simulink model "mpc_model_alignment"  (R2019a)
settings: Solver=FixedStepAuto  StartTime=0.0  StopTime=Tfinal  RelTol=1e-3
values from neighbouring files (symbols this model uses):
  A = [-0.0285 -0.0014; -0.0371 -0.1476]    [model.m]
  AlignmentPeriod = 0.5    [mpc_model_parameters.m]
  DCLINK_Cap = 1000e-12    (= 1e-09)    [mpc_model_parameters.m]    (also in mpc_model_parameters_dual_module.m = 0.001)
  FaultTime = 50    [mpc_model_parameters.m]
  FluxPM = MeanInducedVoltagePeak/(2*pi*100)    [mpc_model_parameters.m]    (also in mpc_model_parameters_dual_module.m)
  Fsw_Alignment = 10000    [mpc_model_parameters.m]
  Inertia = 1e-2    (= 0.01)    [mpc_model_parameters.m]    (also in mpc_model_parameters_dual_module.m)
  Ls = 3.5e-3    (= 0.0035)    [MPC_id_iq.m]    (also in mpc_model_parameters.m = 0.00351; mpc_model_parameters_dual_module.m = 0.00343)
  PolePairs = 10    [mpc_model_parameters.m]    (also in mpc_model_parameters_dual_module.m)
  Rin = 1e-3    (= 0.001)    [mpc_model_parameters.m]    (also in mpc_model_parameters_dual_module.m)
  Rs = 0.531    [Loss_Distribution.m]    (also in MPC_id_iq.m; mpc_model_parameters.m = 0.321; mpc_model_parameters_dual_module.m = 0.539)
  Sampling_time = 1e-6    (= 1e-06)    [mpc_model_parameters.m]    (also in mpc_model_parameters_dual_module.m)
  SpeedRef1 = 0    [mpc_model_parameters.m]    (also in mpc_model_parameters_dual_module.m = 35)
  SpeedRef2 = 50    [mpc_model_parameters.m]    (also in mpc_model_parameters_dual_module.m = 35)
  SpeedRefUpdateTime = 0.5    [mpc_model_parameters.m]    (also in mpc_model_parameters_dual_module.m = 1.75)
  Tload1 = 0    [mpc_model_parameters.m]    (also in mpc_model_parameters_dual_module.m = 30)
  Tload2 = 20    [mpc_model_parameters.m]    (also in mpc_model_parameters_dual_module.m = 63.6619772368)
  TloadUpdateTime = 0.6    [mpc_model_parameters.m]    (also in mpc_model_parameters_dual_module.m = 0.5)
  Vdc = 30    [mpc_model_parameters.m]    (also in mpc_model_parameters_dual_module.m = 40)
  Vin = Vdc + Rin*(Pout/Vdc)    (= 30.0666666667)    [mpc_model_parameters.m]    (also in mpc_model_parameters_dual_module.m = 40.05)
  ViscousFriction = 1e-3    (= 0.001)    [mpc_model_parameters.m]    (also in mpc_model_parameters_dual_module.m)
  whitenoisegain = 0    [mpc_model_parameters.m]
undefined symbols (not defined in the file or in its folder): DiscIntNeverNeededParam
libraries: powerlib x16, dspswit3 x7, simulink x4, powerlib_meascontrol x3, dspstat3 x3, dspsigops x1
settings Model: Creator=hakan  LastModifiedBy=hakan
settings SolverCC: ZeroCrossAlgorithm=Adaptive
settings DebuggingCC: IgnoredZcDiagnostic=none

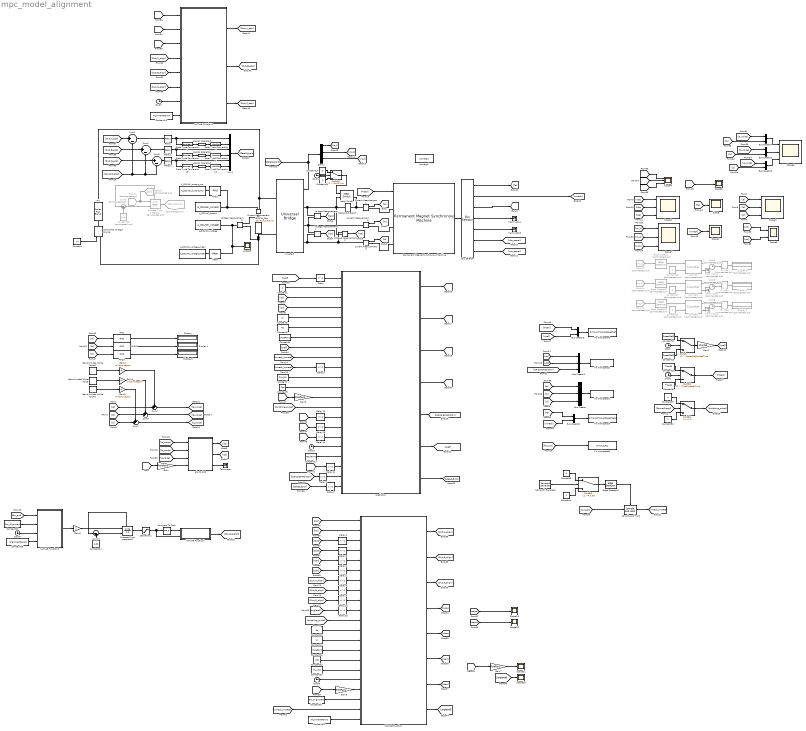
== system mpc_model_alignment ==
  A_DCLINK_current : ToWorkspace  VariableName=A_DCLINK_current  SaveFormat=Structure With Time  SampleTime=-1
  A_DCLINK_current_rms : ToWorkspace  VariableName=A_DCLINK_current_rms  SaveFormat=Structure With Time  SampleTime=-1
  A_DCLINK_voltage : ToWorkspace  VariableName=A_DCLINK_voltage  SaveFormat=Structure With Time  SampleTime=-1
  A_DCLINK_voltage_mean : ToWorkspace  VariableName=A_DCLINK_voltage_mean  SaveFormat=Structure With Time  SampleTime=-1
  Band-Limited White Noise : simulink/Sources/Band-Limited White Noise  Cov=[0.00000002]  Ts=Sampling_time  seed=[23344]  VectorParams1D=off
  Band-Limited White Noise1 : simulink/Sources/Band-Limited White Noise  Cov=[0.00000002]  Ts=Sampling_time  seed=[23343]  VectorParams1D=off
  Band-Limited White Noise2 : simulink/Sources/Band-Limited White Noise  Cov=[0.00000002]  Ts=Sampling_time  seed=[23341]  VectorParams1D=off
  Bus Creator : BusCreator  Inputs=3
  Bus Creator1 : BusCreator  Inputs=3
  Bus Creator{2..6} (5 alike) : BusCreator  Inputs=2
  Bus Selector : BusSelector  OutputSignals=Electromagnetic torque Te (N*m),Rotor speed wm (rad/s),Rotor angle thetam (rad),Stator current is_q (A),Stator current is_d (A),Stator voltage Vs_q (V),Stator voltage Vs_d (V)
  Clock{,1..3,7..9} (7 alike) : Clock
  Clock4 : Clock  Commented=on
  Clock5 : Clock  Commented=on
  Clock6 : Clock  Commented=on
  Compare To Zero : simulink/Logic and Bit Operations/Compare To Zero  relop===  OutDataTypeStr=boolean
  Constant : Constant  Value=Vin
  Constant{1,3,15,29} (4 alike) : Constant  Value=0
  Constant10 : Constant  Value=SpeedRef1
  Constant11 : Constant  Value=SpeedRef2
  Constant12 : Constant  Value=Tload2
  Constant13 : Constant  Value=AlignmentPeriod
  Constant14 : Constant  Value=Ls
  Constant16 : Constant
  Constant17 : Constant  Value=FaultTime
  Constant18 : Constant  Commented=on  Value=0
  Constant19 : Constant  Commented=on  Value=0
  Constant2 : Constant  Value=Ls
  Constant20 : Constant  Commented=on  Value=0
  Constant21 : Constant  Value=Rs
  Constant22 : Constant  Value=PolePairs
  Constant23 : Constant  Value=Vdc
  Constant24 : Constant  Value=1.02
  Constant25 : Constant  Value=AlignmentPeriod
  Constant26 : Constant  Commented=on  Value=1.04
  Constant27 : Constant  Value=Fsw_Alignment
  Constant28 : Constant  Value=AlignmentPeriod
  Constant30 : Constant
  Constant31 : Constant  Value=Fsw_Alignment
  Constant32 : Constant  Value=FluxPM
  Constant4 : Constant
  Constant5 : Constant  Value=Rs
  Constant6 : Constant  Value=PolePairs
  Constant7 : Constant  Value=FluxPM
  Constant8 : Constant  Value=Tload1
  Constant9 : Constant  Value=Vdc
  Controlled Voltage Source : powerlib/Electrical Sources/Controlled Voltage Source  Initialize=on  Source_Type=DC  Amplitude=Vin  Phase=0  Frequency=0  Measurements=None
      settings: SourceProductName=Simscape Electrical
  Counter : dspswit3/Counter  Commented=on  Direction=Up  CountEvent=Rising edge  CounterSize=User defined  MaxCount=9999999999999999999  InitialCount=0  Output=Count and Hit  HitValue=32  ResetInput=on  SamplesPerFrame=1  Ts=1  CntDtype=double  HitDtype=Logical
  Counter1 : dspswit3/Counter  Commented=on  Direction=Up  CountEvent=Rising edge  CounterSize=User defined  MaxCount=9999999999999999999  InitialCount=0  Output=Count and Hit  HitValue=32  ResetInput=on  SamplesPerFrame=1  Ts=1  CntDtype=double  HitDtype=Logical
  Counter2 : dspswit3/Counter  Commented=on  Direction=Up  CountEvent=Rising edge  CounterSize=User defined  MaxCount=9999999999999999999  InitialCount=0  Output=Count and Hit  HitValue=32  ResetInput=on  SamplesPerFrame=1  Ts=1  CntDtype=double  HitDtype=Logical
  Current Measurement{,1..3} (4 alike) : powerlib/Measurements/Current Measurement  PhasorSimulation=off  OutputType=Complex  PSBequivalent=0
      settings: SourceProductName=Simscape Electrical
  DCLINK_Cap : powerlib/Elements/Series RLC Branch  LConnTagsString=__new0  RConnTagsString=__new0  BranchType=C  Resistance=1  Inductance=1e-3  SetiL0=off  InitialCurrent=0  Capacitance=DCLINK_Cap  Setx0=on  InitialVoltage=Vin  Measurements=None
      settings: SourceProductName=Simscape Electrical
  Data Type Conversion10 : DataTypeConversion  OutDataTypeStr=boolean
  Data Type Conversion11 : DataTypeConversion  OutDataTypeStr=double
  Data Type Conversion6 : DataTypeConversion  OutDataTypeStr=boolean
  Data Type Conversion7 : DataTypeConversion  OutDataTypeStr=double
  Data Type Conversion8 : DataTypeConversion  OutDataTypeStr=boolean
  Data Type Conversion9 : DataTypeConversion  OutDataTypeStr=double
  Delay{,1..15} (16 alike) : Delay  DelayLength=1
  Demux : Demux  Outputs=6
  Discrete-Time Integrator : DiscreteIntegrator  Commented=on  ExternalReset=falling  SampleTime=-1  ShowStatePort=on  ICPrevOutput=DiscIntNeverNeededParam  ICPrevScaledInput=DiscIntNeverNeededParam
  Discrete-Time Integrator2 : DiscreteIntegrator  ExternalReset=falling  SampleTime=Sampling_time  UpperSaturationLimit=1  LowerSaturationLimit=0  ShowStatePort=on  ICPrevOutput=DiscIntNeverNeededParam  ICPrevScaledInput=DiscIntNeverNeededParam
  Display : Display
  Display1 : Display  Commented=on
  Display2 : Display  Commented=on
  Display3 : Display  Commented=on
  Display4 : Display
  Display5 : Display
  Divide : Product  Commented=on  Inputs=*/
  Divide1 : Product  Commented=on  Inputs=*/
  Divide2 : Product  Commented=on  Inputs=*/
  Edge Detector : dspswit3/Edge Detector  Commented=on  InputProcessing=Columns as channels (frame based)
      settings: SourceProductName=DSP System Toolbox  SourceProductBaseCode=DS
  Edge Detector1 : dspswit3/Edge Detector  Commented=on  InputProcessing=Columns as channels (frame based)
      settings: SourceProductName=DSP System Toolbox  SourceProductBaseCode=DS
  Edge Detector2 : dspswit3/Edge Detector  Commented=on  InputProcessing=Columns as channels (frame based)
      settings: SourceProductName=DSP System Toolbox  SourceProductBaseCode=DS
  Edge Detector3 : dspswit3/Edge Detector  InputProcessing=Columns as channels (frame based)
      settings: SourceProductName=DSP System Toolbox  SourceProductBaseCode=DS
  From40 : From  Commented=on  GotoTag=va_1
  From41 : From  Commented=on  GotoTag=vb_1
  From42 : From  Commented=on  GotoTag=vc_1
  From72 : From  Commented=on  GotoTag=fsw_out
  Gain{,3,6..7} (4 alike) : Gain  Gain=PolePairs
  Gain1 : Gain  Gain=2*pi/60
  Gain2 : Gain  Gain=whitenoisegain
  Gain4 : Gain  Gain=whitenoisegain
  Gain5 : Gain  Gain=whitenoisegain
  Gain8 : Gain  Gain=2
  Goto29 : Goto  Commented=on  GotoTag=fsw
  Goto9 : Goto  Commented=on  GotoTag=CarrierSignal
  Ideal Switch : powerlib/Power Electronics/Ideal Switch  Ron=0.001  Lon=0  IC=0  Rs=1e5  Cs=inf  Measurements=on
      settings: SourceProductName=Simscape Electrical
  Inverter1 : powerlib/Power Electronics/Universal Bridge  Arms=3  SnubberResistance=1e5  SnubberCapacitance=inf  Device=IGBT / Diodes  Ron=0.65e-3  Lon=0  ForwardVoltages="[  0  0  ]"  ForwardVoltage=0  GTOparameters=[ 10e-6 , 20e-6 ]  IGBTparameters=[ 1e-6 , 2e-6 ]  Measurements=All voltages and currents  Measurements_2=None  converterType=Rectifier
      settings: SourceProductName=Simscape Electrical
  Logical Operator3 : Logic  Operator=NOT  AllPortsSameDT=off  OutDataTypeStr=boolean
  Logical Operator4 : Logic  Operator=NOT  AllPortsSameDT=off  OutDataTypeStr=boolean
  Logical Operator5 : Logic  Operator=NOT  AllPortsSameDT=off  OutDataTypeStr=boolean
  MATLAB Function : MATLAB Function  TreatAsAtomicUnit=on
  MATLAB Function1 : MATLAB Function  TreatAsAtomicUnit=on
  MATLAB Function2 : MATLAB Function  TreatAsAtomicUnit=on
  MATLAB Function3 : MATLAB Function  TreatAsAtomicUnit=on
  Mean : powerlib_meascontrol/Measurements/Mean  Freq=THD_mean_frequency  Vinit=0  Ts=0
      settings: SourceProductName=Simscape Electrical
  Mux4 : Mux  Inputs=6
  Permanent Magnet Synchronous Machine : powerlib/Machines/Permanent Magnet Synchronous Machine  NbPhases=3  FluxDistribution=Sinusoidal  RotorType=Round  MechanicalLoad=Torque Tm  PresetModel=No  ShowDetailedParameters=on  MeasurementBus=off  Resistance=Rs  Inductance=8.5e-3  dqInductances=[3.1e-3,3.6e-3]  La=Ls  MachineConstant=Voltage Constant (V_peak L-L / krpm)  Flux=0.18074  VoltageCst=VoltageConstant  TorqueCst=2.7111  Flat=120  Mechanical=[Inertia ViscousFriction PolePairs 0]  PolePairs=4  InitialConditions=[0*100*2*pi/60,0, 0,0]  InitialConditions5ph=[0 0 0 0 0 0]  TsPowergui=0  TsBlock=-1  RefAngle=90 degrees behind phase A axis (modified Park)
  RMS : dspstat3/RMS  run=off  directionMode=Each column  dimension=1  InputProcessing=Columns as channels (frame based)  reset_popup=None
  RMS1 : powerlib_meascontrol/Measurements/RMS  TrueRMS=on  Freq=Load_Nominal_Freq  RMSInit=10  Ts=0
      settings: SourceProductName=Simscape Electrical
  RMS2 : dspstat3/RMS  run=off  directionMode=Each column  dimension=1  InputProcessing=Columns as channels (frame based)  reset_popup=None
  RMS3 : dspstat3/RMS  run=off  directionMode=Each column  dimension=1  InputProcessing=Columns as channels (frame based)  reset_popup=None
  Relay : Relay
  Relay1 : Relay
  Relay2 : Relay
  Rin : powerlib/Elements/Series RLC Branch  LConnTagsString=__new0  RConnTagsString=__new0  BranchType=R  Resistance=Rin  Inductance=1e-3  SetiL0=off  InitialCurrent=0  Capacitance=1000e-6  Setx0=off  InitialVoltage=0  Measurements=None
      settings: SourceProductName=Simscape Electrical
  Sample and Hold : dspsigops/Sample and Hold  trig=Rising edge  initCond=0  latchinput=off
  Saturation1 : Saturate  UpperLimit=1  LowerLimit=0
  Sawtooth Generator : powerlib_meascontrol/Pulse & Signal Generators/Sawtooth Generator  Freq=100  Phase=180  Ts=0
      settings: SourceProductName=Simscape Electrical
  Scope{,1,5,9..13} (8 alike) : Scope
  Scope{2..4,6..7} (5 alike) : Scope  NumInputPorts=3
  Scope8 : Scope  NumInputPorts=2
  Series RLC Branch : powerlib/Elements/Series RLC Branch  LConnTagsString=__new0  RConnTagsString=__new0  BranchType=R  Resistance=5000  Inductance=1e-3  SetiL0=off  InitialCurrent=0  Capacitance=1e-6  Setx0=off  InitialVoltage=0  Measurements=None
      settings: SourceProductName=Simscape Electrical
  Sum1 : Sum  Inputs=|+-
  Sum10 : Sum  Inputs=|-+
  Sum2 : Sum  Inputs=|+-
  Sum3 : Sum  Commented=on  Inputs=|-+
  Sum4 : Sum  Inputs=++|
  Sum5 : Sum  Inputs=|+-
  Sum6 : Sum  Inputs=++|
  Sum7 : Sum  Inputs=++|
  Switch : Switch  Criteria=u2 > Threshold  Threshold=SpeedRefUpdateTime
  Switch1 : Switch  Criteria=u2 > Threshold  Threshold=TloadUpdateTime
  Switch2 : Switch  Threshold=0.99
  Switch3 : Switch  Criteria=u2 > Threshold  Threshold=FaultTime
  Switch4 : Switch  Criteria=u2 ~= 0
  Terminator : Terminator
  Terminator1 : Terminator  Commented=on
  Terminator2 : Terminator  Commented=on
  Terminator3 : Terminator  Commented=on
  Terminator4 : Terminator
  Terminator5 : Terminator
  To Workspace1 : ToWorkspace  VariableName=Simout_PhaseCurrents_abc  SaveFormat=Timeseries  SampleTime=-1
  To Workspace2 : ToWorkspace  VariableName=Simout_PhaseCurrents_dq  SaveFormat=Timeseries  SampleTime=-1
  To Workspace3 : ToWorkspace  VariableName=Simout_TorqueSpeedMeas  SaveFormat=Timeseries  SampleTime=-1
  To Workspace4 : ToWorkspace  VariableName=Simout_TorqueSpeedRef  SaveFormat=Timeseries  SampleTime=-1
  To Workspace5 : ToWorkspace  VariableName=Simout_Fsw  SaveFormat=Timeseries  SampleTime=-1
  Voltage Measurement{,1..3} (4 alike) : powerlib/Measurements/Voltage Measurement  PhasorSimulation=off  OutputType=Complex  PSBequivalent=0
      settings: SourceProductName=Simscape Electrical
  abc to dq0 : MATLAB Function  TreatAsAtomicUnit=on
  powergui : powerlib/powergui  Priority=1  SimulationMode=Discrete  SampleTime=Sampling_time  frequency=60  Iterations=50  frequencyindice=0  Pbase=100e6  ErrMax=1e-4  UnitsV=kV  UnitsW=MW  buscounter=0  FunctionMessages=off  echomessages=off  EnableUseOfTLC=off  CurrentSourceSwitches=off  DisableSnubberDevices=off  DisableRonSwitches=off  DisableVfSwitches=off  DisplayEquations=off  AutomaticDiscreteSolvers=off  SolverType=Tustin/Backward Euler (TBE)  Interpol=off  ExternalGateDelay=off  methode=off  Ts=100  x0status=blocks  SPID=on  SwTol=0  HookPort=off  NonlinearTolerance=0  nMaxIteration=15  ContinueOnMaxIteration=off  RestoreLinks=warning  ResistiveCurrentMeasurement=off  Frange=[0:2:500]  Ylog=off  Xlog=on  ShowGrid=off  save=off  variable=ZData  structure=0  ZoomFFT=off  StartTime=0.0  cycles=1  DisplayStyle=1  fundamental=60  FreqAxis=off  MaxFrequency=1000  frequencyindicesteady=1  RmsSteady=1  display=off
      settings: SourceProductName=Simscape Electrical
  prediction : MATLAB Function  TreatAsAtomicUnit=on
  wires:
  Voltage Measurement3/1 -> Scope9/1, Mean/1, A_DCLINK_voltage/1
  RMS1/1 -> A_DCLINK_current_rms/1
  Constant/1 -> Controlled Voltage Source/1
  Mean/1 -> A_DCLINK_voltage_mean/1
  Current Measurement/1 -> RMS1/1, A_DCLINK_current/1
  Permanent Magnet Synchronous Machine/1 -> Bus Selector/1
  Bus Selector/1 -> [Te]  "<Electromagnetic torque Te (N*m)>"
  Bus Selector/2 -> [wmech]  "<Rotor speed wm (rad/s)>"
  Current Measurement1/1 -> [Ia]
  Current Measurement2/1 -> [Ib]
  Current Measurement3/1 -> [Ic]
  Bus Selector/3 -> [thetam]  "<Rotor angle thetam (rad)>"
  Bus Selector/4 -> Terminator4/1  "<Stator current is_q (A)>"
  Bus Selector/5 -> Terminator5/1  "<Stator current is_d (A)>"
  [ids] -> prediction/3(IdMeasured)
  [iqs] -> prediction/4(IqMeasured)
  Constant2/1 -> prediction/5(Ls)
  Voltage Measurement/1 -> [Vab]
  Voltage Measurement1/1 -> [Vbc]
  Voltage Measurement2/1 -> [Vca]
  Bus Selector/6 -> [vsq_actual]  "<Stator voltage Vs_q (V)>"
  Bus Selector/7 -> [vsd_actual]  "<Stator voltage Vs_d (V)>"
  [Vca] -> Scope2/3
  [Vbc] -> Scope2/2
  [Vab] -> Scope2/1
  Constant5/1 -> prediction/6(Rs)
  Constant6/1 -> prediction/7(PolePairs)
  [wmech_lowrate] -> prediction/9(ShaftAngularSpeed)
  Constant7/1 -> prediction/11(FluxPM)
  Constant9/1 -> prediction/12(Vdc)
  Gain3/1 -> prediction/13(ElectricalAngle)
  [thetam] -> Gain3/1
  [Tload] -> Permanent Magnet Synchronous Machine/1
  [iqs] -> Bus Creator1/2  "iqs"
  [ids] -> Bus Creator1/1  "ids"
  Constant10/1 -> Switch/3
  Constant11/1 -> Switch/1
  Switch/1 -> Gain1/1
  Clock/1 -> Switch/2
  Clock1/1 -> Switch1/2
  Constant12/1 -> Switch1/1
  Constant8/1 -> Switch1/3
  Switch1/1 -> [Tload]
  Bus Creator/1 -> To Workspace1/1  "Iabc"
  Bus Creator1/1 -> To Workspace2/1  "Idq"
  Bus Creator2/1 -> To Workspace3/1
  Gain1/1 -> [wref]
  [Tload] -> Bus Creator3/1  "Tload"
  [wref] -> Bus Creator3/2  "wref"
  Bus Creator3/1 -> To Workspace4/1
  [switching_pulse] -> prediction/14(InterruptPulse)
  Clock2/1 -> Switch3/2
  Constant15/1 -> Switch3/1
  Constant16/1 -> Switch3/3
  Switch3/1 -> Ideal Switch/1
  Clock3/1 -> prediction/18(SimulationClock)
  Constant17/1 -> prediction/19(FaultOccuranceTime)
  [va_1] -> Scope7/1
  [vb_1] -> Scope7/2
  [vc_1] -> Scope7/3
  Edge Detector/1 -> Counter/1
  Constant18/1 -> Counter/2
  Counter/1 -> Divide/1
  Clock4/1 -> Divide/2
  Divide/1 -> Display2/1
  [Ib] -> Bus Creator/2  "Ib"
  [Ia] -> Bus Creator/1  "Ia"
  [Ic] -> Bus Creator/3  "Ic"
  [Ib] -> Scope3/2  "Ib"
  [Ic] -> Scope3/3  "Ic"
  [Ia] -> Scope3/1  "Ia"
  [iqs] -> Scope8/1  "iqs"
  [ids] -> Scope8/2  "ids"
  Counter/2 -> Terminator1/1
  From40/1 -> Edge Detector/1
  From41/1 -> Edge Detector1/1
  Counter1/2 -> Terminator2/1
  Divide1/1 -> Display1/1
  Clock5/1 -> Divide1/2
  Counter1/1 -> Divide1/1
  Constant19/1 -> Counter1/2
  Edge Detector1/1 -> Counter1/1
  Edge Detector2/1 -> Counter2/1
  Constant20/1 -> Counter2/2
  Counter2/1 -> Divide2/1
  Clock6/1 -> Divide2/2
  Divide2/1 -> Display3/1
  Counter2/2 -> Terminator3/1
  From42/1 -> Edge Detector2/1
  [Te] -> Bus Creator2/1  "Te"
  [wmech] -> Bus Creator2/2  "wmech"
  [Te] -> Scope/1
  [wmech] -> Scope1/1
  prediction/1(DutyA) -> [DutyA]
  prediction/3(DutyC) -> [DutyC]
  prediction/2(DutyB) -> [DutyB]
  [DutyB] -> Scope4/2
  [DutyA] -> Scope4/1
  [DutyC] -> Scope4/3
  Constant26/1 -> Sum3/2
  From72/1 -> Goto29/1, Discrete-Time Integrator/1
  Discrete-Time Integrator/State -> Sum3/1
  Sum3/1 -> Discrete-Time Integrator/2
  Switch4/1 -> [switching_pulse]
  Constant30/1 -> Switch4/3
  Constant29/1 -> Switch4/1
  [GateSignals] -> Inverter1/1, Demux/1
  Demux/1 -> [va_1]
  Demux/3 -> [vb_1]
  prediction/4(FswSelected) -> [fsw_out]
  Delay11/1 -> prediction/20(FswSelected_prev)
  [fsw_out] -> Delay11/1
  [DutyB] -> Delay13/1
  [DutyA] -> Delay12/1
  [DutyC] -> Delay14/1
  Delay13/1 -> prediction/16(DutyB_prev)
  Delay12/1 -> prediction/15(DutyA_prev)
  Delay14/1 -> prediction/17(DutyC_prev)
  Discrete-Time Integrator/1 -> Goto9/1
  [CarrierSignal] -> Switch4/2
  Demux/5 -> [vc_1]
  [IqRipplePrediction] -> Delay1/1
  Delay1/1 -> prediction/21(IqRipplePrediction_prev)
  [CarrierSignal] -> Sum1/2, Sum2/2, Sum5/2
  Logical Operator4/1 -> Data Type Conversion9/1
  [DutyA_app] -> Sum1/1
  Data Type Conversion8/1 -> Logical Operator4/1
  Data Type Conversion10/1 -> Logical Operator5/1
  Relay1/1 -> Data Type Conversion8/1, Mux4/3
  Relay2/1 -> Data Type Conversion10/1, Mux4/5
  Data Type Conversion6/1 -> Logical Operator3/1
  Sum1/1 -> Relay/1
  Data Type Conversion11/1 -> Mux4/6
  [DutyC_app] -> Sum5/1
  Relay/1 -> Mux4/1, Data Type Conversion6/1
  Data Type Conversion9/1 -> Mux4/4
  Sum5/1 -> Relay2/1
  Logical Operator3/1 -> Data Type Conversion7/1
  Logical Operator5/1 -> Data Type Conversion11/1
  Sum2/1 -> Relay1/1
  Mux4/1 -> [GateSignals]
  [DutyB_app] -> Sum2/1
  Data Type Conversion7/1 -> Mux4/2
  [fsw_out] -> Scope5/1
  Discrete-Time Integrator2/State -> Sum10/1
  Gain8/1 -> Discrete-Time Integrator2/1
  Sum10/1 -> Discrete-Time Integrator2/2
  Saturation1/1 -> MATLAB Function1/2(inputwave), Compare To Zero/1
  Constant24/1 -> Sum10/2
  Discrete-Time Integrator2/1 -> Saturation1/1
  Compare To Zero/1 -> MATLAB Function1/1(pulse)
  MATLAB Function1/1(outputwave) -> [CarrierSignal]
  [fsw_out] -> To Workspace5/1
  [IqRipplePrediction] -> Bus Creator1/3  "iqripple"
  Constant1/1 -> prediction/2(idref)
  prediction/5(IqRipplePrediction) -> [IqRipplePrediction]
  Switch2/1 -> Edge Detector3/1
  Edge Detector3/1 -> Sample and Hold/Trigger
  Constant4/1 -> Switch2/3
  Sawtooth Generator/1 -> Switch2/2
  Constant3/1 -> Switch2/1
  [wmech] -> Sample and Hold/1
  Sample and Hold/1 -> [wmech_lowrate]
  [Ia] -> RMS/1
  [Ib] -> RMS2/1
  [Ic] -> RMS3/1
  RMS/1 -> Display/1
  RMS2/1 -> Display4/1
  RMS3/1 -> Display5/1
  abc to dq0/2(iqs) -> [iqs]
  Gain/1 -> abc to dq0/4(ref_frame_position)
  abc to dq0/1(ids) -> [ids]
  abc to dq0/3(i0) -> Terminator/1
  [thetam] -> Gain/1
  Sum4/1 -> [Ia_noise]
  [Ia] -> Sum4/2
  Sum6/1 -> [Ib_noise]
  [Ib] -> Sum6/2
  Sum7/1 -> [Ic_noise]
  [Ic] -> Sum7/2
  Band-Limited White Noise1/1 -> Gain5/1
  Band-Limited White Noise/1 -> Gain4/1
  Band-Limited White Noise2/1 -> Gain2/1
  Gain2/1 -> Sum4/1
  Gain4/1 -> Sum6/1
  Gain5/1 -> Sum7/1
  [Ia_noise] -> abc to dq0/1(ias)
  [Ib_noise] -> abc to dq0/2(ibs)
  [Ic_noise] -> abc to dq0/3(ics)
  [Ia_noise] -> Bus Creator4/1  "Ia_noise"
  [Ia] -> Bus Creator4/2  "Ia"
  [Ib] -> Bus Creator5/2  "Ib"
  [Ib_noise] -> Bus Creator5/1  "Ib_noise"
  [Ic_noise] -> Bus Creator6/1  "Ic_noise"
  [Ic] -> Bus Creator6/2  "Ic"
  Bus Creator5/1 -> Scope6/2
  Bus Creator4/1 -> Scope6/1
  Bus Creator6/1 -> Scope6/3
  prediction/6(iqref) -> [iqref]
  Delay/1 -> prediction/1(iqref_prev)
  [iqref] -> Delay/1
  [wref] -> prediction/8(wref)
  [wmech_lowrate] -> Delay3/1
  prediction/7(Speed_Error) -> [Speed_Error]
  Delay2/1 -> prediction/22(Speed_Error_prev)
  [Speed_Error] -> Delay2/1
  Delay3/1 -> prediction/10(ShaftAngularSpeed_prev)
  MATLAB Function/4(iqapp) -> [iqapp]
  MATLAB Function/5(idapp) -> [idapp]
  MATLAB Function/6(iqerr) -> [iqerr]
  MATLAB Function/7(iderr) -> [iderr]
  [iqapp] -> Delay4/1
  [idapp] -> Delay5/1
  [iqerr] -> Delay6/1
  [iderr] -> Delay7/1
  MATLAB Function/1(DutyA_align) -> [DutyA_align]
  MATLAB Function/2(DutyB_align) -> [DutyB_align]
  MATLAB Function/3(DutyC_align) -> [DutyC_align]
  [DutyA_align] -> Delay8/1
  [DutyB_align] -> Delay9/1
  [DutyC_align] -> Delay10/1
  [switching_pulse] -> MATLAB Function/11(InterruptPulse)
  [iqs] -> MATLAB Function/1(iqmeas)
  [ids] -> MATLAB Function/2(idmeas)
  [DutyA_align] -> MATLAB Function2/4(DutyA_align)
  [DutyC] -> MATLAB Function2/3(DutyC)
  [DutyB] -> MATLAB Function2/2(DutyB)
  [DutyA] -> MATLAB Function2/1(DutyA)
  [DutyB_align] -> MATLAB Function2/5(DutyB_align)
  [DutyC_align] -> MATLAB Function2/6(DutyC_align)
  Clock7/1 -> MATLAB Function2/7(clock)
  Constant13/1 -> MATLAB Function2/8(AlignmentPeriod)
  MATLAB Function2/1(DutyA_app) -> [DutyA_app]
  MATLAB Function2/3(DutyC_app) -> [DutyC_app]
  MATLAB Function2/2(DutyB_app) -> [DutyB_app]
  [thetam] -> Gain6/1
  Constant21/1 -> MATLAB Function/12(Rs)
  Constant14/1 -> MATLAB Function/13(Ls)
  Constant22/1 -> MATLAB Function/14(PolePairs)
  Gain6/1 -> MATLAB Function/18(RotorAngle)
  Constant23/1 -> MATLAB Function/15(Vdc)
  MATLAB Function/8(angleref) -> [angleref]
  [angleref] -> Delay15/1
  Delay4/1 -> MATLAB Function/3(iqapp_prev)
  Delay5/1 -> MATLAB Function/4(idapp_prev)
  Delay6/1 -> MATLAB Function/5(iqerr_prev)
  Delay7/1 -> MATLAB Function/6(iderr_prev)
  Delay8/1 -> MATLAB Function/7(DutyA_align_prev)
  Delay9/1 -> MATLAB Function/8(DutyB_align_prev)
  Delay10/1 -> MATLAB Function/9(DutyC_align_prev)
  Delay15/1 -> MATLAB Function/10(angleref_prev)
  Clock8/1 -> MATLAB Function/17(clock)
  Constant25/1 -> MATLAB Function/21(AlignmentPeriod)
  MATLAB Function3/1(fsw_app) -> Gain8/1
  [fsw_out] -> MATLAB Function3/1(fsw_calculated)
  Constant27/1 -> MATLAB Function3/2(fsw_constant)
  Clock9/1 -> MATLAB Function3/3(clock)
  Constant28/1 -> MATLAB Function3/4(AlignmentPeriod)
  Constant31/1 -> MATLAB Function/19(Fsw_Alignment)
  [wmech_lowrate] -> MATLAB Function/20(wmech)
  Constant32/1 -> MATLAB Function/16(FluxPM)
  [angleref] -> Scope10/1
  [thetam] -> Gain7/1
  Gain7/1 -> Scope11/1
  [iqapp] -> Scope13/1
  [idapp] -> Scope12/1
  connections:
  Rin/LConn1 -- Current Measurement/RConn1 -- Inverter1/RConn1
  Controlled Voltage Source/LConn1 -- Voltage Measurement3/LConn2 -- DCLINK_Cap/RConn1 -- Inverter1/RConn2
  DCLINK_Cap/LConn1 -- Current Measurement/LConn1 -- Voltage Measurement3/LConn1
  Controlled Voltage Source/RConn1 -- Rin/RConn1
  Voltage Measurement2/LConn2 -- Ideal Switch/LConn1 -- Series RLC Branch/LConn1 -- Voltage Measurement/LConn1 -- Inverter1/LConn1
  Current Measurement2/LConn1 -- Voltage Measurement1/LConn1 -- Voltage Measurement/LConn2 -- Inverter1/LConn2
  Inverter1/LConn3 -- Voltage Measurement1/LConn2 -- Voltage Measurement2/LConn1 -- Current Measurement3/LConn1
  Current Measurement3/RConn1 -- Permanent Magnet Synchronous Machine/LConn3
  Permanent Magnet Synchronous Machine/LConn2 -- Current Measurement2/RConn1
  Permanent Magnet Synchronous Machine/LConn1 -- Current Measurement1/RConn1
  Current Measurement1/LConn1 -- Ideal Switch/RConn1 -- Series RLC Branch/RConn1

== matlab function mpc_model_alignment/prediction ==
  data: DutyA output; DutyB output; DutyC output; iqref_prev input; idref input; IdMeasured input; IqMeasured input; Ls input; Rs input; PolePairs input; wref input; ShaftAngularSpeed input; ShaftAngularSpeed_prev input; FluxPM input; Vdc input; ElectricalAngle input; InterruptPulse input; DutyA_prev input; DutyB_prev input; DutyC_prev input; SimulationClock input; FaultOccuranceTime input; FswSelected_prev input; FswSelected output; IqRipplePrediction output; IqRipplePrediction_prev input; iqref output; Speed_Error_prev input; Speed_Error output
function [DutyA, DutyB, DutyC, FswSelected, IqRipplePrediction,iqref,Speed_Error]  = fcn(iqref_prev,idref,IdMeasured, IqMeasured, Ls, Rs,PolePairs,wref, ShaftAngularSpeed,ShaftAngularSpeed_prev, FluxPM,Vdc,ElectricalAngle,InterruptPulse,DutyA_prev, DutyB_prev, DutyC_prev, SimulationClock,FaultOccuranceTime,FswSelected_prev, IqRipplePrediction_prev,Speed_Error_prev)
Ld = Ls;
Lq = Ls;
Iq_Rated = 11.7362; %this is the rated value of the IqMeasured
cost = zeros(1,8);
VdPrediction_1 = zeros(1,8);
VqPrediction_1 = zeros(1,8);
% FswOptions = [5000; 10000; 15000; 20000; 25000; 30000; 35000; 40000];
FswMax = 10000;
FswOptions = 1000:1000:FswMax;
cost = zeros(1,numel(FswOptions));
VdPrediction_1 = zeros(1,numel(FswOptions));
VqPrediction_1 = zeros(1,numel(FswOptions));
VdPrediction_2 = zeros(1,numel(FswOptions));
VqPrediction_2 = zeros(1,numel(FswOptions));
IqRipplePredictionArray_1 = zeros(1,numel(FswOptions));
IqRipplePredictionArray_2 = zeros(1,numel(FswOptions));
VoltageDuring_T1_1 = zeros(1,numel(FswOptions));
VoltageDuring_T2_1 = zeros(1,numel(FswOptions));
VoltageDuring_T0_1 = zeros(1,numel(FswOptions));
VoltageDuring_T1_2 = zeros(1,numel(FswOptions));
VoltageDuring_T2_2 = zeros(1,numel(FswOptions));
VoltageDuring_T0_2 = zeros(1,numel(FswOptions));
MagnitudePrediction_1 = zeros(1,numel(FswOptions));
MagnitudePrediction_2 = zeros(1,numel(FswOptions));

SvpwmT1Prediction_1 =  zeros(1,numel(FswOptions));
SvpwmT2Prediction_1 =  zeros(1,numel(FswOptions));
SvpwmT0Prediction_1 =  zeros(1,numel(FswOptions));

SvpwmT1Prediction_2 =  zeros(1,numel(FswOptions));
SvpwmT2Prediction_2 =  zeros(1,numel(FswOptions));
SvpwmT0Prediction_2 =  zeros(1,numel(FswOptions));

ValfaPrediction_1 = zeros(1,numel(FswOptions)); 
VbetaPrediction_1 = zeros(1,numel(FswOptions)); 
ValfaPrediction_2 = zeros(1,numel(FswOptions)); 
VbetaPrediction_2 = zeros(1,numel(FswOptions)); 
maPrediction_1 = zeros(1,numel(FswOptions)); 
maPrediction_2 = zeros(1,numel(FswOptions));

IqDelta_Prediction_During_T1_1 =  zeros(1,numel(FswOptions));
IqDelta_Prediction_During_T2_1 =  zeros(1,numel(FswOptions));
IqDelta_Prediction_During_T0_1 =  zeros(1,numel(FswOptions));
IqDelta_Prediction_During_T1_2 =  zeros(1,numel(FswOptions));
IqDelta_Prediction_During_T2_2 =  zeros(1,numel(FswOptions));
IqDelta_Prediction_During_T0_2 =  zeros(1,numel(FswOptions));
VoltageVectorAnglePredictionMod_1 = zeros(1,numel(FswOptions));
VoltageVectorAnglePrediction_1 = zeros(1,numel(FswOptions));
VoltageVectorAnglePredictionMod_2 = zeros(1,numel(FswOptions));
VoltageVectorAnglePrediction_2 = zeros(1,numel(FswOptions));

IdPrediction_1_array = zeros(1,numel(FswOptions));
IqPrediction_1_array = zeros(1,numel(FswOptions));
IdPrediction_2_array = zeros(1,numel(FswOptions));
IqPrediction_2_array = zeros(1,numel(FswOptions));

MinimumCostValue = 1e20;
MinimumCostIndex = -1;

IqRippleCoeff = 100000;
IqRefCoeff = 10000;
IdRefCoeff = 15;
FswCoeff = 1250;
Iq_1_Method1 = 0;
Id_1_Method1 = 0;
Iq_2_Method1 = 0;
Id_2_Method1 = 0;
Kp = 0.35;
Ki = 10;
Ts_PI = 1/40000;
% y = y_prev + Kp*(u-u_prev)+Ts/2*Ki*(u+u_prev);
if(InterruptPulse==1)
    Speed_Error =  wref-ShaftAngularSpeed;
    
    iqref = iqref_prev + Kp*(Speed_Error-Speed_Error_prev)+Ts_PI/2*Ki*((Speed_Error+Speed_Error_prev));
%     if(iqref>(2*Iq_Rated))
%         iqref = 2*Iq_Rated;
%     end
%     if(iqref<(-2*Iq_Rated))
%         iqref = -2*Iq_Rated;
%     end
    if(abs(iqref)>(2*Iq_Rated))
        if(iqref>0)
            iqref = (2*Iq_Rated);
        else
            iqref = -(2*Iq_Rated);
        end
    end
    for i = 1:numel(FswOptions)
        %% first prediction
        VdPrediction_1(i) = Rs*IdMeasured + Ld*FswOptions(i)*(idref-IdMeasured)-PolePairs*ShaftAngularSpeed*Lq*IqMeasured;
        VqPrediction_1(i) = Rs*IqMeasured + Lq*FswOptions(i)*(iqref-IqMeasured)+PolePairs*ShaftAngularSpeed*(Ld*IdMeasured+FluxPM);
        
%         MagnitudePrediction_1(i) = sqrt(VdPrediction_1(i)^2+VqPrediction_1(i)^2);
%         
%         ValfaPrediction_1(i) = sin(ElectricalAngle)*VdPrediction_1(i)+cos(ElectricalAngle)*VqPrediction_1(i);
%         VbetaPrediction_1(i) =-cos(ElectricalAngle)*VdPrediction_1(i)+sin(ElectricalAngle)*VqPrediction_1(i);     
%         
%         VoltageVectorAnglePrediction_1(i) = atan2(VbetaPrediction_1(i),ValfaPrediction_1(i))+4*pi;
%         VoltageVectorAnglePredictionMod_1(i) = mod(VoltageVectorAnglePrediction_1(i),pi/3);
%         
%         maPrediction_1(i) = MagnitudePrediction_1(i)/(Vdc/sqrt(3));
%         
%         SvpwmT1Prediction_1(i) = (1/FswOptions(i))*maPrediction_1(i)*sin(pi/3-VoltageVectorAnglePredictionMod_1(i));
%         SvpwmT2Prediction_1(i) = (1/FswOptions(i))*maPrediction_1(i)*sin(VoltageVectorAnglePredictionMod_1(i));
%         SvpwmT0Prediction_1(i) = (1/FswOptions(i))-SvpwmT1Prediction_1(i)-SvpwmT2Prediction_1(i);        
%         
%         VoltageDuring_T1_1(i) = 2/3*Vdc-MagnitudePrediction_1(i);
%         VoltageDuring_T2_1(i) = 2/3*Vdc-MagnitudePrediction_1(i);
%         VoltageDuring_T0_1(i) = -MagnitudePrediction_1(i);
%         
%         IqDelta_Prediction_During_T1_1(i) = VoltageDuring_T1_1(i)*SvpwmT1Prediction_1(i)/Ls;
%         IqDelta_Prediction_During_T2_1(i) = VoltageDuring_T2_1(i)*SvpwmT2Prediction_1(i)/Ls;
%         IqDelta_Prediction_During_T0_1(i) = -VoltageDuring_T0_1(i)*SvpwmT0Prediction_1(i)/Ls;
%         
%         IqRipplePredictionArray_1(i) = IqDelta_Prediction_During_T1_1(i)+IqDelta_Prediction_During_T2_1(i)+IqDelta_Prediction_During_T0_1(i);
        
        %predict the future output
        IdPrediction_1 = IdMeasured + (1/FswOptions(i))*(VdPrediction_1(i)/Ld-Rs/Ld*IdMeasured+Lq/Ld*PolePairs*ShaftAngularSpeed*IqMeasured);
        IqPrediction_1 = IqMeasured + (1/FswOptions(i))*(VqPrediction_1(i)/Lq-Rs/Lq*IqMeasured-Ld/Lq*PolePairs*ShaftAngularSpeed*IdMeasured-FluxPM*PolePairs*ShaftAngularSpeed/Lq);
        TePrediction_1 = 1.5*PolePairs*(FluxPM*IqPrediction_1+0*(Ld-Lq)*IdPrediction_1*IqPrediction_1); % reluctance torque component is multiplied by 0, since it caused unreasonable torque values.
                
        IdPrediction_1_array(i) = IdPrediction_1;
        IqPrediction_1_array(i) = IqPrediction_1;
        
        %% second prediction
        VdPrediction_2(i) = Rs*IdPrediction_1 + Ld*FswOptions(i)*(idref-IdMeasured)-PolePairs*ShaftAngularSpeed*Lq*IqPrediction_1;
        VqPrediction_2(i) = Rs*IqPrediction_1 + Lq*FswOptions(i)*(iqref-IqMeasured)+PolePairs*ShaftAngularSpeed*(Ld*IdPrediction_1+FluxPM);        
        
        MagnitudePrediction_2(i) = sqrt(VdPrediction_2(i)^2+VqPrediction_2(i)^2);
        
        ValfaPrediction_2(i) = sin(ElectricalAngle)*VdPrediction_2(i)+cos(ElectricalAngle)*VqPrediction_2(i);
        VbetaPrediction_2(i) =-cos(ElectricalAngle)*VdPrediction_2(i)+sin(ElectricalAngle)*VqPrediction_2(i);      
        
        VoltageVectorAnglePrediction_2(i) = atan2(VbetaPrediction_2(i),ValfaPrediction_2(i))+4*pi;
        VoltageVectorAnglePredictionMod_2(i) = mod(VoltageVectorAnglePrediction_2(i),pi/3);   
        
        maPrediction_2(i) = MagnitudePrediction_2(i)/(Vdc/sqrt(3)); 
        
        SvpwmT1Prediction_2(i) = (1/FswOptions(i))*maPrediction_2(i)*sin(pi/3-VoltageVectorAnglePredictionMod_2(i));
        SvpwmT2Prediction_2(i) = (1/FswOptions(i))*maPrediction_2(i)*sin(VoltageVectorAnglePredictionMod_2(i));
        SvpwmT0Prediction_2(i) = (1/FswOptions(i))-SvpwmT1Prediction_2(i)-SvpwmT2Prediction_2(i); 
        
        VoltageDuring_T1_2(i) = 2/3*Vdc-MagnitudePrediction_2(i);
        VoltageDuring_T2_2(i) = 2/3*Vdc-MagnitudePrediction_2(i);
        VoltageDuring_T0_2(i) = -MagnitudePrediction_2(i);
        
        IqDelta_Prediction_During_T1_2(i) = VoltageDuring_T1_2(i)*SvpwmT1Prediction_2(i)/Ls;
        IqDelta_Prediction_During_T2_2(i) = VoltageDuring_T2_2(i)*SvpwmT2Prediction_2(i)/Ls;
        IqDelta_Prediction_During_T0_2(i) = -VoltageDuring_T0_2(i)*SvpwmT0Prediction_2(i)/Ls;        
        
        IqRipplePredictionArray_2(i) = IqDelta_Prediction_During_T1_2(i)+IqDelta_Prediction_During_T2_2(i)+IqDelta_Prediction_During_T0_2(i);
        
        IdPrediction_2 = IdPrediction_1 + (1/FswOptions(i))*(VdPrediction_2(i)/Ld-Rs/Ld*IdPrediction_1+Lq/Ld*PolePairs*ShaftAngularSpeed*IqPrediction_1);
        IqPrediction_2 = IqPrediction_1 + (1/FswOptions(i))*(VqPrediction_2(i)/Lq-Rs/Lq*IqPrediction_1-Ld/Lq*PolePairs*ShaftAngularSpeed*IdPrediction_1-FluxPM*PolePairs*ShaftAngularSpeed/Lq);                
        
        IdPrediction_2_array(i) = IdPrediction_2;
        IqPrediction_2_array(i) = IqPrediction_2;
        
        %% calculate the cost
        if(abs(IqPrediction_1)>30)||(abs(TePrediction_1)>50)
            ProtectionConstant = inf;
        else
            ProtectionConstant = 0;
        end
%         cost(i) = (IqRipplePredictionArray_1(i)/Iq_Rated)^2*IqRippleCoeff+IqRefCoeff*((iqref-IqPrediction_1)/Iq_Rated)^2+((idref-IdPrediction_1)/Iq_Rated)^2*IdRefCoeff+ProtectionConstant+FswOptions(i)/FswMax*FswCoeff;%+IqRipplePrediction_prev^2*100000000;
        cost(i) = (IqRipplePredictionArray_2(i)/Iq_Rated)^2*IqRippleCoeff+IqRefCoeff*((iqref-IqPrediction_2)/Iq_Rated)^2+((idref-IdPrediction_2)/Iq_Rated)^2*IdRefCoeff+ProtectionConstant+FswOptions(i)/FswMax*FswCoeff;%+IqRipplePrediction_prev^2*100000000;
        if(cost(i)<MinimumCostValue)
            MinimumCostValue = cost(i);
            MinimumCostIndex = i;
        end
        
    end
    
%     [CostMinVal, MinimumCostIndex] = min(cost);
    
    DutyA = 0;
    DutyB = 0;
    DutyC = 0;
    VdsOptimum_1 = VdPrediction_2(MinimumCostIndex);
    VqsOptimum_1 = VqPrediction_2(MinimumCostIndex);
    FswSelected = FswOptions(MinimumCostIndex);
    
    Iq_1_Method1 = IqPrediction_1_array(MinimumCostIndex);
    Id_1_Method1 = IdPrediction_1_array(MinimumCostIndex);

    Iq_2_Method1 = IqPrediction_2_array(MinimumCostIndex);
    Id_2_Method1 = IdPrediction_2_array(MinimumCostIndex);
    
    VoltageVectorAngleOptimum = VoltageVectorAnglePrediction_2(MinimumCostIndex);
    TswSelected = 1/FswSelected;

    
    Svpwm_T1 = SvpwmT1Prediction_2(MinimumCostIndex);
    Svpwm_T2 = SvpwmT2Prediction_2(MinimumCostIndex);
    Svpwm_T0 = SvpwmT0Prediction_2(MinimumCostIndex);
    
    IqRipplePrediction = IqRipplePredictionArray_2(MinimumCostIndex);
    
    if (mod(VoltageVectorAngleOptimum, 2*pi)<=pi/3)&&(mod(VoltageVectorAngleOptimum, 2*pi)>=0)  % sector 1
        DutyA = (Svpwm_T1+Svpwm_T2+Svpwm_T0/2)/TswSelected;
        DutyB = (Svpwm_T2+Svpwm_T0/2)/TswSelected;
        DutyC = (Svpwm_T0/2)/TswSelected;
%         sectornumber = 1;
        return;
    end
    if (mod(VoltageVectorAngleOptimum, 2*pi)<=2*pi/3)&&(mod(VoltageVectorAngleOptimum, 2*pi)>=pi/3)  % sector 2
        DutyA = (Svpwm_T1+Svpwm_T0/2)/TswSelected;
        DutyB = (Svpwm_T1+Svpwm_T2+Svpwm_T0/2)/TswSelected;
        DutyC = (Svpwm_T0/2)/TswSelected;
%         sectornumber = 2;
        return;
    end
    if (mod(VoltageVectorAngleOptimum, 2*pi)<=pi)&&(mod(VoltageVectorAngleOptimum, 2*pi)>=2*pi/3)  % sector 3
        if(mod(VoltageVectorAngleOptimum, pi)==0)
            DutyA = (Svpwm_T0/2)/TswSelected;
            DutyB = (Svpwm_T1+Svpwm_T0/2)/TswSelected;
            DutyC = (Svpwm_T1+Svpwm_T2+Svpwm_T0/2)/TswSelected;
        else
            DutyA = (Svpwm_T0/2)/TswSelected;
            DutyB = (Svpwm_T1+Svpwm_T2+Svpwm_T0/2)/TswSelected;
            DutyC = (Svpwm_T2+Svpwm_T0/2)/TswSelected;
        end
%         sectornumber = 3;
        return;
    end
    if (mod(VoltageVectorAngleOptimum, 2*pi)<=4*pi/3)&&(mod(VoltageVectorAngleOptimum, 2*pi)>=pi)  % sector 4
        DutyA = (Svpwm_T0/2)/TswSelected;
        DutyB = (Svpwm_T1+Svpwm_T0/2)/TswSelected;
        DutyC = (Svpwm_T1+Svpwm_T2+Svpwm_T0/2)/TswSelected;
%         sectornumber = 4;
        return;
    end
    if (mod(VoltageVectorAngleOptimum, 2*pi)<=5*pi/3)&&(mod(VoltageVectorAngleOptimum, 2*pi)>=4*pi/3)  % sector 5
        DutyA = (Svpwm_T2+Svpwm_T0/2)/TswSelected;
        DutyB = (Svpwm_T0/2)/TswSelected;
        DutyC = (Svpwm_T1+Svpwm_T2+Svpwm_T0/2)/TswSelected;
%         sectornumber = 5;
        return;
    end
    if (mod(VoltageVectorAngleOptimum, 2*pi)<=2*pi)&&(mod(VoltageVectorAngleOptimum, 2*pi)>=5*pi/3)  % sector 6
        DutyA = (Svpwm_T1+Svpwm_T2+Svpwm_T0/2)/TswSelected;
        DutyB = (Svpwm_T0/2)/TswSelected;
        DutyC = (Svpwm_T1+Svpwm_T0/2)/TswSelected;
%         sectornumber = 6;
        return;
    end
    
else %switching pulse
    iqref = iqref_prev;
    Speed_Error = Speed_Error_prev;
    FswSelected = FswSelected_prev;
    DutyA = DutyA_prev;
    DutyB = DutyB_prev;
    DutyC = DutyC_prev;
    IqRipplePrediction = IqRipplePrediction_prev;
end

== matlab function mpc_model_alignment/MATLAB Function ==
  data: iqmeas input; idmeas input; iqapp_prev input; idapp_prev input; iqerr_prev input; iderr_prev input; DutyA_align_prev input; DutyA_align output; DutyB_align output; DutyC_align output; DutyB_align_prev input; DutyC_align_prev input; angleref_prev input; InterruptPulse input; iqapp output; idapp output; iqerr output; iderr output; Rs input; Ls input; PolePairs input; Vdc input; FluxPM input; clock input; RotorAngle input; Fsw_Alignment input; wmech input; angleref output; AlignmentPeriod input
function [DutyA_align, DutyB_align, DutyC_align,iqapp,idapp,iqerr,iderr,angleref] = fcn(iqmeas,idmeas,iqapp_prev,idapp_prev,iqerr_prev,iderr_prev,DutyA_align_prev, DutyB_align_prev, DutyC_align_prev,angleref_prev,InterruptPulse,Rs,Ls,PolePairs,Vdc,FluxPM, clock,RotorAngle,Fsw_Alignment, wmech, AlignmentPeriod)
iqrated = 11.7362;
Ld = Ls;
Lq = Ls;
iqref = 0;
idref = 11.7362/2;
Ts_PI = 1/40000;
Kp = 0.35;
Ki = 10;
ElectricalAngle = 0;
DutyA_align = 0;
DutyB_align = 0;
DutyC_align = 0;
if((InterruptPulse==1)&&(clock<AlignmentPeriod))
    
    angleref = RotorAngle;
    
    iqerr = iqref-iqmeas;
    iqapp = iqapp_prev + Kp*(iqerr - iqerr_prev)+Ts_PI/2*Ki*(iqerr+iqerr_prev);
    if(abs(iqapp)>(2*iqrated))
        if(iqapp>0)
            iqapp = (2*iqrated);
        else
            iqapp = -(2*iqrated);
        end
    end    
    
    iderr = idref-idmeas;
    idapp = idapp_prev + Kp*(iderr - iderr_prev)+Ts_PI/2*Ki*(iderr+iderr_prev);
    if(abs(idapp)>(2*iqrated))
        if(idapp>0)
            idapp = (2*iqrated);
        else
            idapp = -(2*iqrated);
        end
    end     
    
    vd = Rs*idmeas + Ld*Fsw_Alignment*(idref-idmeas)-PolePairs*wmech*Lq*iqmeas;
    vq = Rs*iqmeas + Lq*Fsw_Alignment*(iqref-iqmeas)+PolePairs*wmech*(Ld*idmeas+FluxPM);
    
    magnitude = sqrt(vd^2+vq^2);
      
    valfa = sin(ElectricalAngle)*vd+cos(ElectricalAngle)*vq;
    vbeta =-cos(ElectricalAngle)*vd+sin(ElectricalAngle)*vq;     
    
    voltagevectorangle = atan2(vbeta,valfa);
    voltagevectorangle_mod = mod(voltagevectorangle,pi/3);
    
    ma = magnitude/(Vdc/sqrt(3));
    
    Svpwm_T1 = (1/Fsw_Alignment)*ma*sin(pi/3-voltagevectorangle_mod);
    Svpwm_T2 = (1/Fsw_Alignment)*ma*sin(voltagevectorangle_mod);
    Svpwm_T0 = (1/Fsw_Alignment)-Svpwm_T1-Svpwm_T2;
    
    Ts = 1/Fsw_Alignment;
    
    
    if (mod(voltagevectorangle, 2*pi)<=pi/3)&&(mod(voltagevectorangle, 2*pi)>=0)  % sector 1
        DutyA_align = (Svpwm_T1+Svpwm_T2+Svpwm_T0/2)/Ts;
        DutyB_align = (Svpwm_T2+Svpwm_T0/2)/Ts;
        DutyC_align = (Svpwm_T0/2)/Ts;
%         sectornumber = 1;
        return;
    end
    if (mod(voltagevectorangle, 2*pi)<=2*pi/3)&&(mod(voltagevectorangle, 2*pi)>=pi/3)  % sector 2
        DutyA_align = (Svpwm_T1+Svpwm_T0/2)/Ts;
        DutyB_align = (Svpwm_T1+Svpwm_T2+Svpwm_T0/2)/Ts;
        DutyC_align = (Svpwm_T0/2)/Ts;
%         sectornumber = 2;
        return;
    end
    if (mod(voltagevectorangle, 2*pi)<=pi)&&(mod(voltagevectorangle, 2*pi)>=2*pi/3)  % sector 3
        if(mod(voltagevectorangle, pi)==0)
            DutyA_align = (Svpwm_T0/2)/Ts;
            DutyB_align = (Svpwm_T1+Svpwm_T0/2)/Ts;
            DutyC_align = (Svpwm_T1+Svpwm_T2+Svpwm_T0/2)/Ts;
        else
            DutyA_align = (Svpwm_T0/2)/Ts;
            DutyB_align = (Svpwm_T1+Svpwm_T2+Svpwm_T0/2)/Ts;
            DutyC_align = (Svpwm_T2+Svpwm_T0/2)/Ts;
        end
%         sectornumber = 3;
        return;
    end
    if (mod(voltagevectorangle, 2*pi)<=4*pi/3)&&(mod(voltagevectorangle, 2*pi)>=pi)  % sector 4
        DutyA_align = (Svpwm_T0/2)/Ts;
        DutyB_align = (Svpwm_T1+Svpwm_T0/2)/Ts;
        DutyC_align = (Svpwm_T1+Svpwm_T2+Svpwm_T0/2)/Ts;
%         sectornumber = 4;
        return;
    end
    if (mod(voltagevectorangle, 2*pi)<=5*pi/3)&&(mod(voltagevectorangle, 2*pi)>=4*pi/3)  % sector 5
        DutyA_align = (Svpwm_T2+Svpwm_T0/2)/Ts;
        DutyB_align = (Svpwm_T0/2)/Ts;
        DutyC_align = (Svpwm_T1+Svpwm_T2+Svpwm_T0/2)/Ts;
%         sectornumber = 5;
        return;
    end
    if (mod(voltagevectorangle, 2*pi)<=2*pi)&&(mod(voltagevectorangle, 2*pi)>=5*pi/3)  % sector 6
        DutyA_align = (Svpwm_T1+Svpwm_T2+Svpwm_T0/2)/Ts;
        DutyB_align = (Svpwm_T0/2)/Ts;
        DutyC_align = (Svpwm_T1+Svpwm_T0/2)/Ts;
%         sectornumber = 6;
        return;
    end    
    
    
else
    iqerr = iqerr_prev;
    iderr = iderr_prev;
    iqapp = iqapp_prev;
    idapp = idapp_prev;    
    DutyA_align = DutyA_align_prev;
    DutyB_align = DutyB_align_prev;
    DutyC_align = DutyC_align_prev;   
    angleref = angleref_prev;

end

== matlab function mpc_model_alignment/MATLAB Function2 ==
  data: DutyA input; DutyA_app output; DutyB input; DutyC input; DutyA_align input; DutyB_align input; DutyC_align input; DutyB_app output; DutyC_app output; clock input; AlignmentPeriod input
function [DutyA_app, DutyB_app, DutyC_app] = fcn(DutyA, DutyB, DutyC, DutyA_align, DutyB_align, DutyC_align,clock,AlignmentPeriod)

if(clock>AlignmentPeriod)
    DutyA_app = DutyA;
    DutyB_app = DutyB;
    DutyC_app = DutyC;    
else
    DutyA_app = DutyA_align;
    DutyB_app = DutyB_align;
    DutyC_app = DutyC_align;        
end

== matlab function mpc_model_alignment/abc to dq0 ==
  data: ids output; iqs output; ias input; ibs input; ics input; ref_frame_position input; i0 output
function [ids,iqs,i0 ]  = fcn(ias,ibs,ics,ref_frame_position)





ids = 2/3*(ias*sin(ref_frame_position)+ibs*sin(ref_frame_position-2*pi/3)+ics*sin(ref_frame_position+2*pi/3));
iqs =  2/3*(ias*cos(ref_frame_position)+ibs*cos(ref_frame_position-2*pi/3)+ics*cos(ref_frame_position+2*pi/3));
i0 = 2/3*1/2*(ias+ibs+ics);
% iqs = (vqs-fluxlinkage_qs_derivative-ref_frame_velocity*fluxlinkage_ds)/rs;
% ids = (vds-fluxlinkage_ds_derivative+ref_frame_velocity*fluxlinkage_qs)/rs;

== matlab function mpc_model_alignment/MATLAB Function3 ==
  data: fsw_calculated input; fsw_app output; fsw_constant input; clock input; AlignmentPeriod input
function fsw_app  = fcn(fsw_calculated, fsw_constant,clock,AlignmentPeriod)

if(clock>AlignmentPeriod)
    fsw_app = fsw_calculated;    
else
    fsw_app = fsw_constant;       
end

== matlab function mpc_model_alignment/MATLAB Function1 ==
  data: pulse input; inputwave input; outputwave output
function outputwave  = fcn(pulse, inputwave)

persistent state

if isempty(state)
state = 0;
end

if(pulse==1)
    state = state +1;
end

if(mod(state,2)==1)
    outputwave = inputwave;
    return;
end
if(mod(state,2)==0)
    outputwave = 1-inputwave;
    return;
end

outputwave = 5;
